simulink model "ThrustCommand_Solution"  (R2025b)
settings: Solver=FixedStepDiscrete  StartTime=0.0  StopTime=inf  FixedStep=1e-5  RelTol=1e-3
libraries: simulink x2
settings Model: Creator=diego  LastModifiedBy=diego

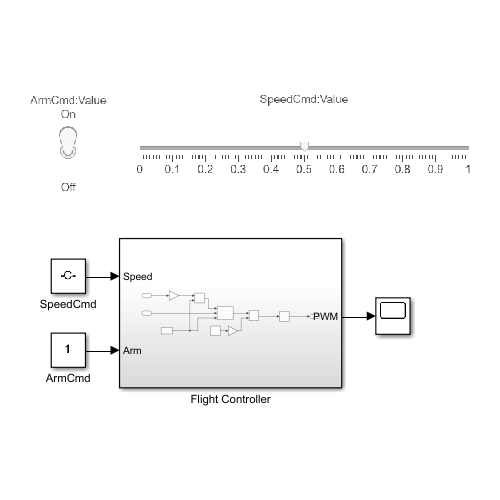
[thumbnail: Simulink's stored preview of the top-level diagram]
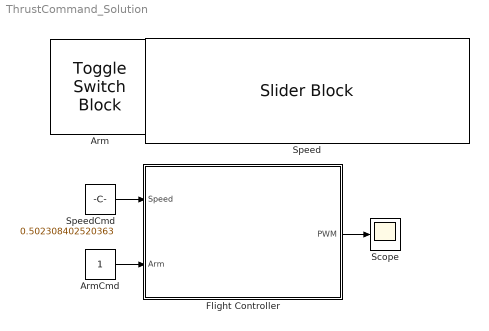
== system ThrustCommand_Solution ==
  "Arm " : ToggleSwitchBlock
  ArmCmd : Constant
  Flight Controller : Subsystem
  Scope : Scope
      settings: TimeSpan=0.05  ActiveDisplayYMinimum=0  ActiveDisplayYMaximum=1
  Speed : SliderBlock  ScaleMax=1  TickInterval=0.1
  SpeedCmd : Constant  Value=0.502308402520363
  wires:
  Flight Controller/1(PWM) -> Scope/1
  SpeedCmd/1 -> Flight Controller/1(Speed)
  ArmCmd/1 -> Flight Controller/2(Arm)

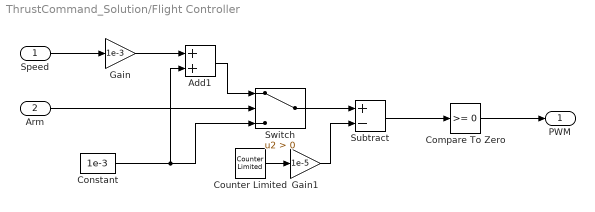
== system ThrustCommand_Solution/Flight Controller ==
  Speed : Inport
  Arm : Inport  Port=2
  Add1 : Sum
  Compare To Zero : simulink/Logic and Bit Operations/Compare To Zero  relop=>=  OutDataTypeStr=boolean
  Constant : Constant  Value=1e-3
  Counter Limited : simulink/Sources/Counter Limited  uplimit=1999  tsamp=-1
  Gain : Gain  Gain=1e-3
  Gain1 : Gain  Gain=1e-5
  Subtract : Sum  Inputs=+-
  Switch : Switch  Criteria=u2 > Threshold  SaturateOnIntegerOverflow=off  InputSameDT=off
  PWM : Outport
  wires:
  Constant/1 -> Switch/3, Add1/2
  Add1/1 -> Switch/1
  Compare To Zero/1 -> PWM/1
  Switch/1 -> Subtract/1
  Counter Limited/1 -> Gain1/1
  Subtract/1 -> Compare To Zero/1
  Gain/1 -> Add1/1
  Speed/1 -> Gain/1
  Arm/1 -> Switch/2
  Gain1/1 -> Subtract/2
